simulink model "EJ3_240623_Cd"  (R2021a)
settings: Solver=ode8  StartTime=0.0  StopTime=30  FixedStep=Ts  RelTol=1e-3
values from neighbouring files (symbols this model uses):
  Ts = 0.1    [Linealizacion.m]
  ue = 1    [Linealizacion.m]
  x1e = 2    [Linealizacion.m]
  x2e = 1    [Linealizacion.m]
  ye = 1    [Linealizacion.m]
libraries: cstblocks x1
settings Model: Creator=aghersin  LastModifiedBy=Santiago
settings SolverCC: AlgebraicLoopSolver=TrustRegion
settings DataIOCC: ReturnWorkspaceOutputs=off
settings OptimizationCC: LifeSpan=inf
settings DebuggingCC: SFExecutionAtInitializationDiag=none  SFMachineParentedDataDiag=warning  ArithmeticOperatorsInVariantConditions=warning
settings SFSimCC: SimUseLocalCustomCode=off  CustomCodeUndefinedFunction=UseInterfaceOnly
settings RTWCC: RTWUseLocalCustomCode=off
settings CodeAppCC: StateflowObjectComments=on

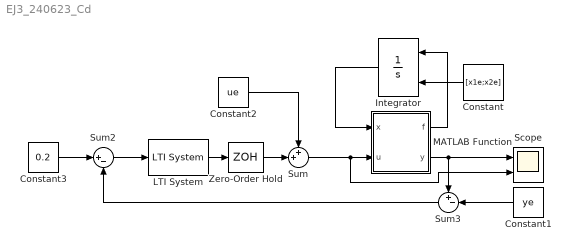
== system EJ3_240623_Cd ==
  Constant : Constant  Value=[x1e;x2e]  VectorParams1D=off
  Constant1 : Constant  Value=ye
  Constant2 : Constant  Value=ue
  Constant3 : Constant  Value=0.2
  Integrator : Integrator  InitialConditionSource=external
  LTI System : cstblocks/LTI System  sys=C_digital  IC=[]
  MATLAB Function : MATLAB Function  TreatAsAtomicUnit=on
  Scope : Scope  NumInputPorts=2
  Sum : Sum  Inputs=++|
  Sum2 : Sum  Inputs=|+-
  Sum3 : Sum  Inputs=+-|
  Zero-Order Hold : ZeroOrderHold  SampleTime=Ts
  wires:
  LTI System/1 -> Zero-Order Hold/1
  Constant2/1 -> Sum/1
  Sum2/1 -> LTI System/1
  MATLAB Function/1(f) -> Integrator/1
  Constant3/1 -> Sum2/1
  Sum3/1 -> Sum2/2
  Constant/1 -> Integrator/2
  MATLAB Function/2(y) -> Sum3/1, Scope/1
  Constant1/1 -> Sum3/2
  Zero-Order Hold/1 -> Sum/2
  Sum/1 -> Scope/2, MATLAB Function/2(u)
  Integrator/1 -> MATLAB Function/1(x)

== matlab function EJ3_240623_Cd/MATLAB Function ==
  data: x input; u input; f output; y output
function [f,y] = fcn(x,u)

f1 = -sqrt(abs(x(1) - x(2))) + u;
f2 = sqrt(abs(x(1) - x(2))) - sqrt(x(2));

f=[f1; f2];

y=x(2);
